simulink model "threephaseACACcontrollerdelta"  (R2021a)
settings: Solver=VariableStepAuto  StartTime=0.0  StopTime=10.0  RelTol=1e-3
libraries: spsThyristorLib x6, spsVoltageMeasurementLib x3, spsMultimeterLib x2, powerlib_extras x1, spsThreePhaseSeriesRLCBranchLib x1, spsThreePhaseVIMeasurementLib x1, spsThreePhaseSourceLib x1, spspowerguiLib x1
settings Model: Creator=User  LastModifiedBy=User

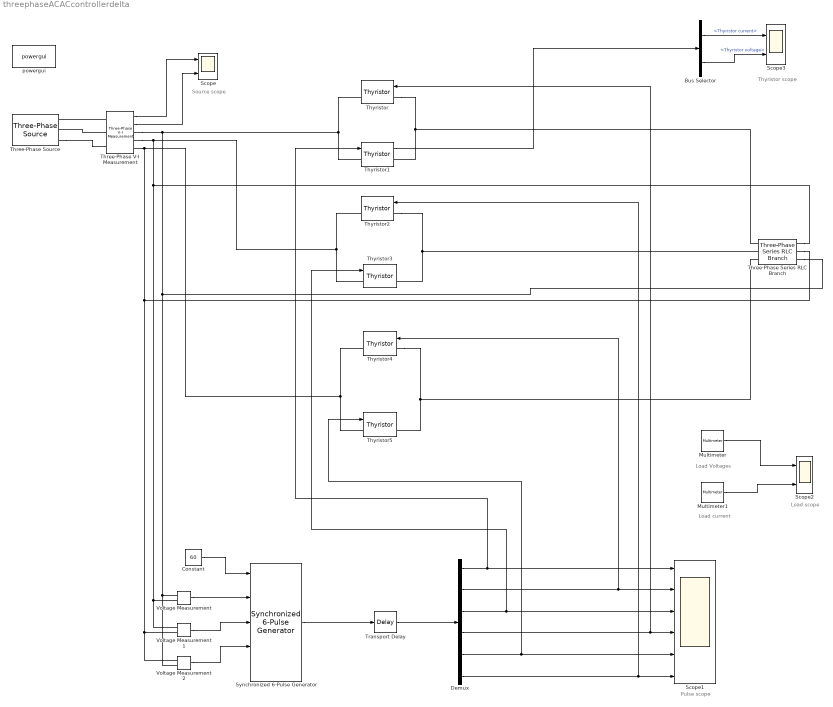
== system threephaseACACcontrollerdelta ==
  note: Load current
  note: Load scope
  note: Pulse scope
  note: Load Voltages
  note: Source scope
  note: Thyristor scope
  Bus Selector : BusSelector  OutputSignals=Thyristor current,Thyristor voltage
  Constant : Constant  Value=60
  Demux : Demux  Outputs=6
  Multimeter : spsMultimeterLib/Multimeter  PhasorSimulation=off  OutputType=Complex  sel=[1 2 3]  L=6  Gain=[1 1 1]  yselected={'Ub1: Three-Phase Series RLC Branch','Ub2: Three-Phase Series RLC Branch','Ub3: Three-Phase Series RLC Branch'};  PSBOutputType=1  PSBequivalent=0  AxesSetting=[0,0.1,-100,100]  Display=0  SavedBlockNames=-11
  Multimeter1 : spsMultimeterLib/Multimeter  PhasorSimulation=off  OutputType=Complex  sel=[4 5 6]  L=6  Gain=[1 1 1]  yselected={'Ib1: Three-Phase Series RLC Branch','Ib2: Three-Phase Series RLC Branch','Ib3: Three-Phase Series RLC Branch'};  PSBOutputType=1  PSBequivalent=0  AxesSetting=[0,0.1,-100,100]  Display=0  SavedBlockNames=-11
  Scope : Scope  NumInputPorts=2
  Scope1 : Scope  NumInputPorts=6
  Scope2 : Scope  NumInputPorts=2
  Scope3 : Scope  NumInputPorts=2
  Synchronized 6-Pulse Generator : powerlib_extras/Control  Blocks/Synchronized 6-Pulse Generator  freq=50  pwidth=10  Double_Pulse=on
      settings: SourceProductBaseCode=PS
  Three-Phase Series RLC Branch : spsThreePhaseSeriesRLCBranchLib/Three-Phase Series RLC Branch  LConnTagsString=A|B|C  RConnTagsString=A|B|C  BranchType=RL  Resistance=10  Inductance=0.01  Capacitance=1e-6  Measurements=Branch voltages and currents
  Three-Phase V-I Measurement : spsThreePhaseVIMeasurementLib/Three-Phase V-I Measurement  VoltageMeasurement=phase-to-ground  SetLabelV=off  LabelV=Vabc  Vpu=off  VpuLL=off  CurrentMeasurement=yes  SetLabelI=off  LabelI=Iabc  Ipu=off  Pbase=100e6  Vbase=500e3  OutputType=Complex  PhasorSimulation=off  PSBequivalent=0
  Three-Phase Source : spsThreePhaseSourceLib/Three-Phase Source  InternalConnection=Yg  VoltagePhases=off  Voltage=380  PhaseAngle=0  Voltage_phases=[25e3 25e3 25e3]/sqrt(3)  PhaseAngles_phases=[0 -120 +120]  Frequency=50  NonIdealSource=on  SpecifyImpedance=off  Resistance=0  Inductance=0  ShortCircuitLevel=100e6  BaseVoltage=25e3  XRratio=7  BusType=swing  Pref=10e3  Qref=0  Prefabc=[10e3, 10e3, 10e3]  Qrefabc=[0, 0, 0]  Qmin=-inf  Qmax=inf
  Thyristor{,1..5} (6 alike) : spsThyristorLib/Thyristor  Ron=0.001  Lon=0  Vf=0.8  IC=0  Rs=500  Cs=250e-9  Measurements=on
  Transport Delay : TransportDelay  DelayTime=330*0.02/360
  Voltage Measurement : spsVoltageMeasurementLib/Voltage Measurement  PhasorSimulation=off  OutputType=Complex  PSBequivalent=0
  Voltage Measurement1 : spsVoltageMeasurementLib/Voltage Measurement  PhasorSimulation=off  OutputType=Complex  PSBequivalent=0
  Voltage Measurement2 : spsVoltageMeasurementLib/Voltage Measurement  PhasorSimulation=off  OutputType=Complex  PSBequivalent=0
  powergui : spspowerguiLib/powergui  Priority=1  SimulationMode=Continuous  SampleTime=50e-6  frequency=60  Iterations=50  frequencyindice=50  Pbase=100e6  ErrMax=1e-4  UnitsV=kV  UnitsW=MW  buscounter=0  FunctionMessages=off  echomessages=off  EnableUseOfTLC=off  CurrentSourceSwitches=off  DisableSnubberDevices=off  DisableRonSwitches=off  DisableVfSwitches=off  DisplayEquations=off  AutomaticDiscreteSolvers=off  SolverType=Tustin/Backward Euler (TBE)  Interpol=off  ExternalGateDelay=off  methode=off  Ts=100  x0status=blocks  SPID=on  SwTol=0  HookPort=off  NonlinearTolerance=1e-4  nMaxIteration=100  ContinueOnMaxIteration=off  RestoreLinks=warning  ResistiveCurrentMeasurement=off  Frange=[0:2:500]  Ylog=off  Xlog=on  ShowGrid=off  save=off  variable=ZData  structure=0  ZoomFFT=off  StartTime=0.0  cycles=1  DisplayStyle=1  fundamental=60  FreqAxis=off  MaxFrequency=1000  frequencyindicesteady=1  RmsSteady=1  display=off
  wires:
  Voltage Measurement/1 -> Synchronized 6-Pulse Generator/2
  Demux/4 -> Thyristor/1, Scope1/4
  Voltage Measurement1/1 -> Synchronized 6-Pulse Generator/3
  Thyristor1/1 -> Bus Selector/1
  Demux/5 -> Scope1/5, Thyristor5/1
  Demux/2 -> Thyristor4/1, Scope1/2
  Bus Selector/1 -> Scope3/1  "<Thyristor current>"
  Multimeter1/1 -> Scope2/2
  Transport Delay/1 -> Demux/1
  Three-Phase V-I Measurement/1 -> Scope/1
  Multimeter/1 -> Scope2/1
  Demux/6 -> Thyristor2/1, Scope1/6
  Synchronized 6-Pulse Generator/1 -> Transport Delay/1
  Demux/3 -> Scope1/3, Thyristor3/1
  Demux/1 -> Scope1/1, Thyristor1/1
  Bus Selector/2 -> Scope3/2  "<Thyristor voltage>"
  Constant/1 -> Synchronized 6-Pulse Generator/1
  Three-Phase V-I Measurement/2 -> Scope/2
  Voltage Measurement2/1 -> Synchronized 6-Pulse Generator/4
  connections:
  Three-Phase V-I Measurement/RConn2 -- Three-Phase Series RLC Branch/RConn1 -- Voltage Measurement1/LConn1 -- Voltage Measurement/LConn2 -- Thyristor2/RConn1 -- Thyristor3/LConn1
  Thyristor3/RConn1 -- Thyristor2/LConn1 -- Three-Phase Series RLC Branch/LConn2
  Thyristor5/RConn1 -- Thyristor4/LConn1 -- Three-Phase Series RLC Branch/LConn3
  Voltage Measurement1/LConn2 -- Thyristor4/RConn1 -- Thyristor5/LConn1 -- Three-Phase V-I Measurement/RConn3 -- Three-Phase Series RLC Branch/RConn2 -- Voltage Measurement2/LConn1
  Three-Phase V-I Measurement/RConn1 -- Three-Phase Series RLC Branch/RConn3 -- Voltage Measurement/LConn1 -- Voltage Measurement2/LConn2 -- Thyristor/RConn1 -- Thyristor1/LConn1
  Three-Phase Series RLC Branch/LConn1 -- Thyristor/LConn1 -- Thyristor1/RConn1
  Three-Phase Source/RConn3 -- Three-Phase V-I Measurement/LConn3
  Three-Phase V-I Measurement/LConn2 -- Three-Phase Source/RConn2
  Three-Phase V-I Measurement/LConn1 -- Three-Phase Source/RConn1
